simulink model "testjump"  (R2019b)
settings: Solver=VariableStepAuto  StartTime=0.0  StopTime=10.0  RelTol=1e-3
libraries: dspsrcs4 x1
settings Model: Creator=cwhipp  LastModifiedBy=cwhipp

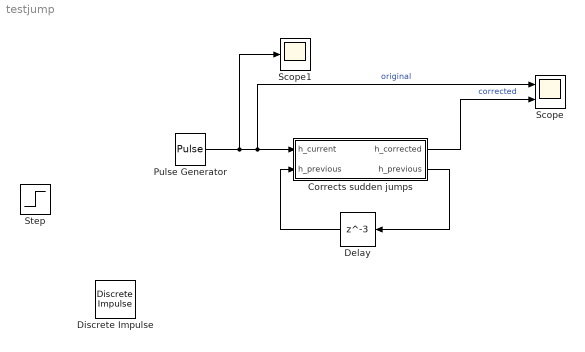
== system testjump ==
  Corrects sudden jumps : MATLAB Function  TreatAsAtomicUnit=on
  Delay : Delay  DelayLength=3  InitialCondition=zeros(1,3)  SampleTime=0.005
  Discrete Impulse : dspsrcs4/Discrete  Impulse  Delay=10  SampleTime=1  FrameSample=1  OutputFrames=off  dataType=double  isSigned=on  wordLen=16  udDataType=sfix(16)  fracBitsMode=Best precision  numFracBits=15  OutDataTypeStr=double  LastOutDataTypeStr=double
  Pulse Generator : DiscretePulseGenerator  PulseType=Time based  Amplitude=3  PulseWidth=0.01
  Scope : Scope  NumInputPorts=2
  Scope1 : Scope
  Step : Step  After=10  SampleTime=0.005
  wires:
  Delay/1 -> Corrects sudden jumps/2("h_previous ")
  Corrects sudden jumps/2(h_previous) -> Delay/1
  Pulse Generator/1 -> Scope1/1, Scope/1, Corrects sudden jumps/1(h_current)  "original"
  Corrects sudden jumps/1(h_corrected) -> Scope/2  "corrected"

== matlab function testjump/Corrects sudden jumps ==
  data: h_current input; h_corrected output; h_previous input; h_previous output
function [h_corrected, h_previous] = fcn(h_current, h_previous)

diffthreshold = 1;

previous_average = mean(h_previous);

h_change = abs(h_current-previous_average);

if(h_change > diffthreshold)
    h_corrected = h_previous(1);
else
    h_corrected = h_current;
end

h_previous = [h_current; h_previous(1:end-1)];
